simulink model "eVTOL"  (R2025b)
settings: Solver=ode45  StartTime=0.0  StopTime=7  MaxStep=1e-4  RelTol=1e-3
InitFcn:
  | load('inner_controller_design.mat')
  | load('outer_controller_design.mat')
  | load('speed_controller_design.mat')
  | load('position_controller_design.mat')
  | load('tita_controller_design.mat')
values from neighbouring files (symbols this model uses):
  b = 1e-4    (= 0.0001)    [LE_final.m]    (also in outer_controller_design.mat)
  denC = [Kc*Tcontrolador,1]    [LI_final.m]    (also in inner_controller_design.mat = [0.0127388535032 1])
  J_motor = 0.01*(0.432^2)*2    (= 0.00373248)    [LE_final.m]    (also in outer_controller_design.mat)
  J_xz = 3.25    [angular_speed_controller_design.mat]    (also in tita_controller_design.mat = 2.16666666667)
  K_pos_den = [1 2.17655923708]    [position_controller_design.mat]
  K_pos_num = [0 1.57913670417]    [position_controller_design.mat]
  Ke = 1 / Kv_rad_per_V    (= 0.0347247148564)    [LE_final.m]    (also in outer_controller_design.mat)
  KF = 0.000504745724606    [speed_controller_design.mat]
  Ki = K * z    [LE_final.m]    (also in outer_controller_design.mat = 13312.7522358)
  Kp = K    [LE_final.m]    (also in outer_controller_design.mat = 52.8005114253)
  kQ = alpha_rpm * rpm2rad^-2    (= 1.07603097028e-05)    [LE_final.m]    (also in outer_controller_design.mat)
  Kt = 1*Ke    (= 0.0347247148564)    [LE_final.m]    (also in outer_controller_design.mat)
  Ktita_den = [1 61.1449635422]    [tita_controller_design.mat]
  Ktita_num = [1557.79440274 15875.2136603]    [tita_controller_design.mat]
  Kv_den = 1    [speed_controller_design.mat]
  Kv_num = 65.3451271947    [speed_controller_design.mat]
  l = 0.3    [speed_controller_design.mat]
  l_palanca = 0.4    [tita_controller_design.mat]
  La = 0.0004    [LI_final.m]    (also in inner_controller_design.mat)
  m = 13    [speed_controller_design.mat]
  numC = [Tcontrolador,1]    [LI_final.m]    (also in inner_controller_design.mat = [0.00398089171975 1])
  Ra = 0.066    [LI_final.m]    (also in inner_controller_design.mat)
libraries: slpidlib x5, simulink_extras x4
(part 1 of 2)
settings Model: PacingRate=0.089000  Creator=Allan  LastModifiedBy=Allan

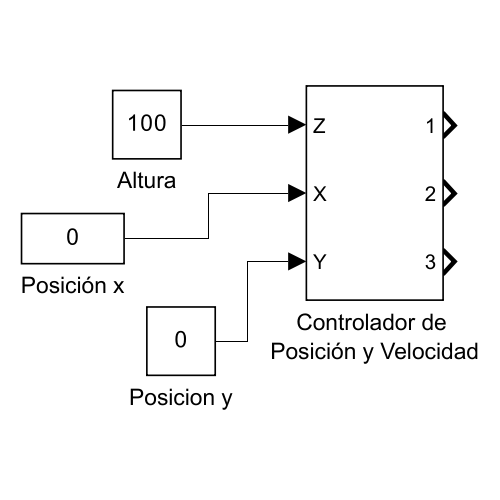
[thumbnail: Simulink's stored preview of the top-level diagram]
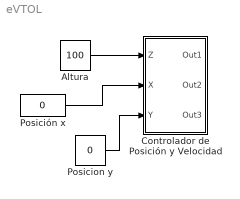
== system eVTOL ==
  Altura : Constant  Value=100
  Controlador de Posición y Velocidad : Subsystem
  Posicion y : Constant  Value=0
  Posición x : Constant  Value=0
  wires:
  Altura/1 -> Controlador de Posición y Velocidad/1(Z)
  Posición x/1 -> Controlador de Posición y Velocidad/2(X)
  Posicion y/1 -> Controlador de Posición y Velocidad/3(Y)

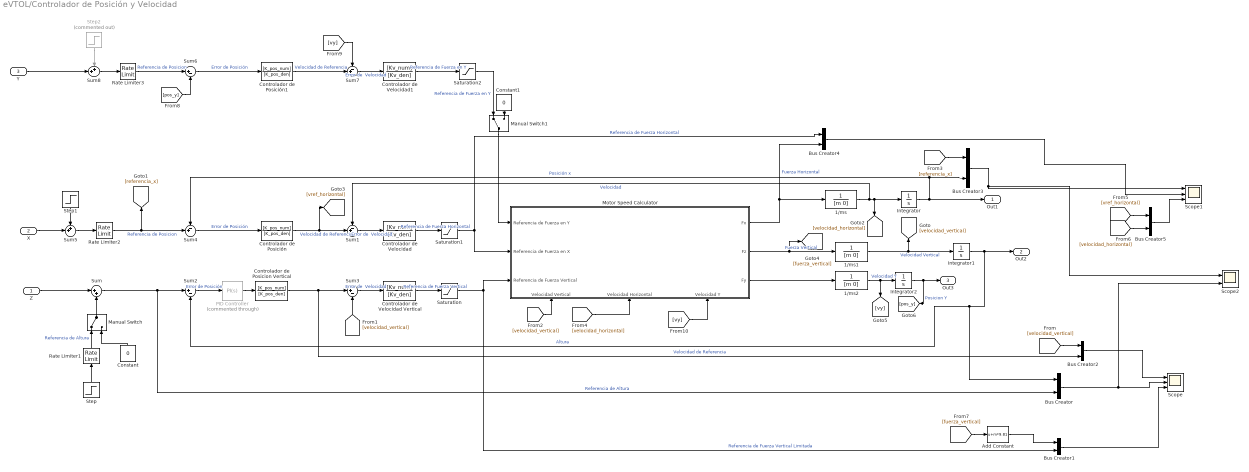
== system eVTOL/Controlador de Posición y Velocidad ==
  Z : Inport
  X : Inport  Port=2
  Y : Inport  Port=3
  1/ms : TransferFcn  Denominator=[m 0]
  1/ms1 : TransferFcn  Denominator=[m 0]
  1/ms2 : TransferFcn  Denominator=[m 0]
  Add Constant : Bias  Bias=m*9.81  SaturateOnIntegerOverflow=off
  Bus Creator{,1..5} (6 alike) : BusCreator  Inputs=2
  Constant : Constant  Value=0
  Constant1 : Constant  Value=0
  Controlador de Velocidad : TransferFcn  Numerator=[Kv_num]  Denominator=[Kv_den]
  Controlador de Velocidad1 : TransferFcn  Numerator=[Kv_num]  Denominator=[Kv_den]
  Controlador de Posicion Vertical : TransferFcn  Numerator=[K_pos_num]  Denominator=[K_pos_den]
  Controlador de Posición : TransferFcn  Numerator=[K_pos_num]  Denominator=[K_pos_den]
  Controlador de Posición1 : TransferFcn  Numerator=[K_pos_num]  Denominator=[K_pos_den]
  Controlador de Velocidad Vertical : TransferFcn  Numerator=[Kv_num]  Denominator=[Kv_den]
  Integrator : Integrator
  Integrator1 : Integrator  InitialCondition=100
  Integrator2 : Integrator
  Manual Switch : ManualSwitch
  Manual Switch1 : ManualSwitch
  Motor Speed Calculator : Subsystem
      settings: PortSchema="{\"entries\":[{\"content\":{\"sides\":[{\"content\":{\"connectorIds\":[\"In1\",\"In2\",\"In3\"]},\"type\":\"ConnectorPlacement.EquallySpacedRectSide\",\"uuid\":\"7b759047-1fb7-4341-8a14-a3cb95641d34\"},{\"content\":{\"connectorIds\":[\"Out1\",\"Out2\",\"Out3\"],\"side\":\"RIGHT\"},\"type\":\"ConnectorPlacement.EquallySpacedRectSide\",\"uuid\":\"2a3f944b-70ea-4cc6-8a8c-2d0c7e75b016\"},{\"content\":{\"side\":\"TOP\"},\"type\":\"ConnectorPlacement.EquallySpacedRectSide\",\"uuid\":\"5d8f49a3-64b1-4126-af97-ef65cef9ee4f\"},{\"content\":{\"connectorIds\":[\"In4\",\"In5\",\"In6\"],\"side\":\"BOTTOM\"},\"type\":\"ConnectorPlacement.EquallySpacedRectSide\",\"uuid\":\"3a67fbcc-1ab1-41a0-8583-aff8280d6eaa\"}]},\"type\":\"ConnectorPlacement.EquallySpacedConnector\",\"uuid\":\"910e2bb6-9332-485b-94fd-5d2df90e8b0c\"}],\"packageUris\":[\"http://schema.mathworks.com/mf0/Connector/R2020b\"],\"version\":\"1.0\"}"
  PID Controller : slpidlib/PID Controller  Commented=through  Controller=PI  Form=Parallel  TimeDomain=Continuous-time  UseExternalTs=off  SampleTime=-1  IntegratorMethod=Forward Euler  FilterMethod=Forward Euler  ControllerParametersSource=internal  P=4.353  I=6.317  UseKiTs=off  D=0  UseExternalDerivativeSource=off  N=100  UseFilter=on  TunerSelectOption=Transfer Function Based (PID Tuner App)  InitialConditionSource=internal  InitialConditionForIntegrator=0  InitialConditionForFilter=0  DifferentiatorICPrevScaledInput=0  ExternalReset=none  TrackingMode=off  Kt=1  LimitOutput=on  SatLimitsSource=internal  UpperSaturationLimit=inf  LowerSaturationLimit=-inf  LinearizeAsGain=on  AntiWindupMode=clamping  Kb=1  LimitIntegrator=off  UpperIntegratorSaturationLimit=inf  LowerIntegratorSaturationLimit=-inf  POutMin=[]  POutMax=[]  IOutMin=[]  IOutMax=[]  DOutMin=[]  DOutMax=[]  NOutMin=[]  NOutMax=[]  SumOutMin=[]  SumOutMax=[]  SaturationOutMin=[]  SaturationOutMax=[]  PParamMin=[]  PParamMax=[]  IParamMin=[]  IParamMax=[]  DParamMin=[]  DParamMax=[]  NParamMin=[]  NParamMax=[]  KbParamMin=[]  KbParamMax=[]  KtParamMin=[]  KtParamMax=[]  KbOutMin=[]  KbOutMax=[]  KtOutMin=[]  KtOutMax=[]  IntegratorOutMin=[]  IntegratorOutMax=[]  FilterOutMin=[]  FilterOutMax=[]  SumI1OutMin=[]  SumI1OutMax=[]  SumI2OutMin=[]  SumI2OutMax=[]  SumI3OutMin=[]  SumI3OutMax=[]  SumI4OutMin=[]  SumI4OutMax=[]  SumDOutMin=[]  SumDOutMax=[]  DifferentiatorOutMin=[]  DifferentiatorOutMax=[]  FilterDiffOutCoefMin=[]  FilterDiffOutCoefMax=[]  ReciprocalOutMin=[]  ReciprocalOutMax=[]  SumDenOutMin=[]  SumDenOutMax=[]  SumNumOutMin=[]  SumNumOutMax=[]  DivideOutMin=[]  DivideOutMax=[]  UdiffTsProdOutMin=[]  UdiffTsProdOutMax=[]  NTsProdOutMin=[]  NTsProdOutMax=[]  UintegralTsProdOutMin=[]  UintegralTsProdOutMax=[]  UngainTsProdOutMin=[]  UngainTsProdOutMax=[]  ClampingZeroOutDataTypeStr=Inherit: Inherit via back propagation  ClampingZeroOutMin=[]  ClampingZeroOutMax=[]  FilterDenConstantOutDataTypeStr=Inherit: Inherit via back propagation  FilterDenConstantOutMin=[]  FilterDenConstantOutMax=[]  PCopyOutDataTypeStr=Inherit: Inherit via back propagation  PCopyOutMin=[]  PCopyOutMax=[]  NCopyOutDataTypeStr=Inherit: Inherit via back propagation  NCopyOutMin=[]  NCopyOutMax=[]  IntegratorContinuousStateAttributes=''  IntegratorStateMustResolveToSignalObject=off  IntegratorRTWStateStorageClass=Auto  FilterContinuousStateAttributes=''  FilterStateMustResolveToSignalObject=off  FilterRTWStateStorageClass=Auto  ParallelPVariant=InternalParameters  IdealPVariant=Disabled  IVariant=InternalParameters  DVariant=Disabled  IntegratorVariant=Continuous  SatVariant=Enabled  AWVariant=ContClampingParallel  PCopyVariant=Disabled  TRVariant=Disabled  FdbkBlocksVariant=Forward  IdealPFdbkVariant=Disabled  SatFdbkVariant=Disabled  DerivativeFilterVariant=Disabled  NVariant=Disabled  NCopyVariant=Disabled_SignalSpec  FilterICVariant=Disabled  IntegratorICVariant=InternalICs  ExternalResetVariant=Disabled  TRSumVariant=Passthrough  SumFdbkVariant=Disabled  SumVariant=Sum_PI  TsampFilterVariant=InternalTs  TsampNgainVariant=Passthrough  TsampIntegralVariant=Disabled_SignalSpec  ExternalSaturationOutDataTypeStr=Inherit: Same as second input  DerivativeSourceVariant=Disabled  PreIntVariant=InternalPreInt
  Rate Limiter1 : RateLimiter  RisingSlewLimit=5  FallingSlewLimit=-5  SampleTimeMode=inherited  LinearizeAsGain=off
  Rate Limiter2 : RateLimiter  RisingSlewLimit=5  FallingSlewLimit=-5  SampleTimeMode=inherited  LinearizeAsGain=off
  Rate Limiter3 : RateLimiter  RisingSlewLimit=2  FallingSlewLimit=-2  SampleTimeMode=inherited  LinearizeAsGain=off
  Saturation : Saturate  UpperLimit=1.6*m*9.81  LowerLimit=0.4*m*9.81
  Saturation1 : Saturate  UpperLimit=0.2*m*9.81  LowerLimit=-0.2*m*9.81
  Saturation2 : Saturate  UpperLimit=0.5*m*9.81  LowerLimit=-0.5*m*9.81
  Scope : Scope  NumInputPorts=3
      settings: ActiveDisplayYMinimum=97.035286958696958  ActiveDisplayYMaximum=105.88496811570035  DataLoggingVariableName=ScopeData2
  Scope1 : Scope  NumInputPorts=3
      settings: ActiveDisplayYMinimum=-1.0400119613662664  ActiveDisplayYMaximum=9.3601076522964  DataLoggingVariableName=ScopeData6
  Scope2 : Scope  NumInputPorts=2
      settings: ActiveDisplayYMinimum=-0.12959032213957208  ActiveDisplayYMaximum=1.1663128992561491  DataLoggingVariableName=ScopeData7
  Step : Step  After=5  SampleTime=0
  Step1 : Step  SampleTime=0
  Step2 : Step  Commented=on  After=4  SampleTime=0
  Sum : Sum  Inputs=|++
  Sum1 : Sum  Inputs=-+|
  Sum2 : Sum  Inputs=|+-
  Sum3 : Sum  Inputs=|+-
  Sum4 : Sum  Inputs=-+|
  Sum5 : Sum  Inputs=++|
  Sum6 : Sum  Inputs=|+-
  Sum7 : Sum  Inputs=-+|
  Sum8 : Sum  Inputs=++|
  Out1 : Outport
  Out2 : Outport  Port=2
  Out3 : Outport  Port=3
  wires:
  Controlador de Posición/1 -> [vref_horizontal], Sum1/2  "Velocidad de Referencia"
  Sum4/1 -> Controlador de Posición/1  "Error de Posición"
  Sum1/1 -> Controlador de Velocidad/1  "Error de  Velocidad"
  1/ms/1 -> [velocidad_horizontal], Integrator/1, Sum1/1  "Velocidad"
  Integrator/1 -> Out1/1, Sum4/1, Bus Creator3/2  "Posición x"
  Integrator1/1 -> Sum2/2, Bus Creator/1, Out2/1  "Altura"
  Sum3/1 -> Controlador de Velocidad Vertical/1  "Error de  Velocidad"
  Sum2/1 -> PID Controller/1  "Error de Posición"
  1/ms1/1 -> [velocidad_vertical], Integrator1/1  "Velocidad Vertical"
  Controlador de Posicion Vertical/1 -> Sum3/1, Bus Creator2/2  "Velocidad de Referencia"
  Controlador de Velocidad/1 -> Saturation1/1  "Referencia de Fuerza Horizontal"
  Rate Limiter2/1 -> Sum4/2, [referencia_x]  "Referencia de Posicion"
  Sum/1 -> Bus Creator/2, Sum2/1  "Referencia de Altura"
  Motor Speed Calculator/1(Fx) -> Bus Creator4/2, 1/ms/1  "Fuerza Horizontal"
  Motor Speed Calculator/2(Fz) -> [fuerza_vertical], 1/ms1/1  "Fuerza Vertical"
  Step/1 -> Rate Limiter1/1
  Z/1 -> Sum/1
  Bus Creator/1 -> Scope2/2, Scope/2
  Bus Creator1/1 -> Scope/3
  Saturation/1 -> Motor Speed Calculator/3(Referencia de Fuerza Vertical), Bus Creator1/2  "Referencia de Fuerza Vertical Limitada"
  Saturation1/1 -> Bus Creator4/1, Motor Speed Calculator/2(Referencia de Fuerza en X)  "Referencia de Fuerza Horizontal"
  Bus Creator2/1 -> Scope/1
  Controlador de Velocidad Vertical/1 -> Saturation/1  "Referencia de Fuerza Vertical"
  [velocidad_vertical] -> Bus Creator2/1
  [velocidad_vertical] -> Sum3/2
  [velocidad_vertical] -> Motor Speed Calculator/4(Velocidad Vertical)
  Add Constant/1 -> Bus Creator1/1
  PID Controller/1 -> Controlador de Posicion Vertical/1
  Step1/1 -> Sum5/1
  X/1 -> Sum5/2
  Sum5/1 -> Rate Limiter2/1
  [referencia_x] -> Bus Creator3/1
  Bus Creator3/1 -> Scope2/1, Scope1/1
  [velocidad_horizontal] -> Motor Speed Calculator/5(Velocidad Horizontal)
  Bus Creator4/1 -> Scope1/2
  [velocidad_horizontal] -> Bus Creator5/2
  [vref_horizontal] -> Bus Creator5/1
  Bus Creator5/1 -> Scope1/3
  Sum6/1 -> Controlador de Posición1/1  "Error de Posición"
  Controlador de Velocidad1/1 -> Saturation2/1  "Referencia de Fuerza en Y"
  Controlador de Posición1/1 -> Sum7/2  "Velocidad de Referencia"
  Sum7/1 -> Controlador de Velocidad1/1  "Error de  Velocidad"
  [fuerza_vertical] -> Add Constant/1
  Motor Speed Calculator/3(Fy) -> 1/ms2/1
  1/ms2/1 -> Integrator2/1, [vy]  "Velocidad Y"
  Integrator2/1 -> [pos_y], Out3/1  "Posicion Y"
  [pos_y] -> Sum6/2
  [vy] -> Sum7/1
  Step2/1 -> Sum8/1
  Sum8/1 -> Rate Limiter3/1
  Y/1 -> Sum8/2
  Rate Limiter3/1 -> Sum6/1  "Referencia de Posicion"
  [vy] -> Motor Speed Calculator/6(Velocidad Y)
  Rate Limiter1/1 -> Manual Switch/1  "Referencia de Altura"
  Manual Switch/1 -> Sum/2
  Constant/1 -> Manual Switch/2
  Saturation2/1 -> Manual Switch1/1  "Referencia de Fuerza en Y"
  Manual Switch1/1 -> Motor Speed Calculator/1(Referencia de Fuerza en Y)
  Constant1/1 -> Manual Switch1/2

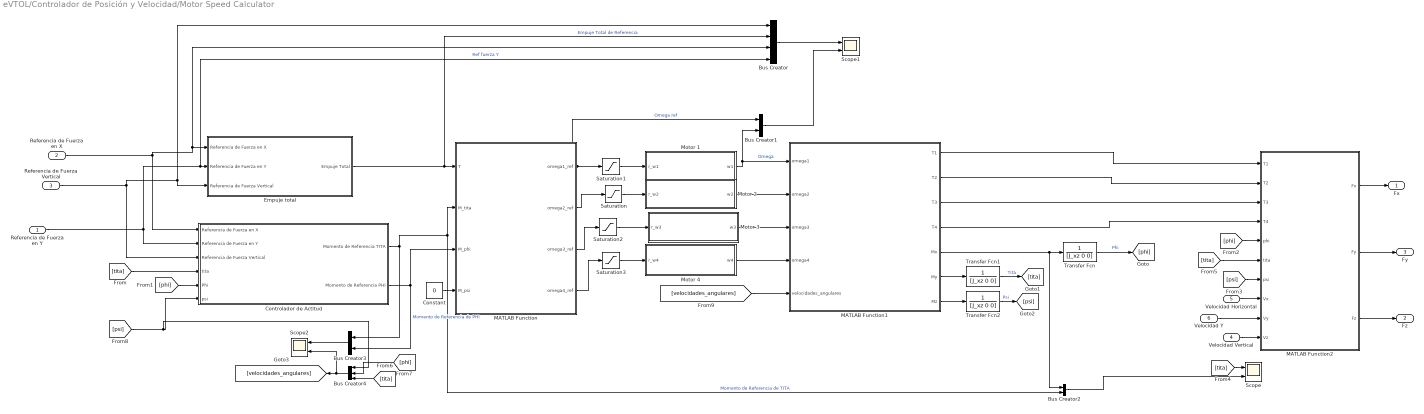
== system eVTOL/Controlador de Posición y Velocidad/Motor Speed Calculator ==
  Referencia de Fuerza en Y : Inport
  Referencia de Fuerza en X : Inport  Port=2
  Referencia de Fuerza Vertical : Inport  Port=3
  Velocidad Vertical : Inport  Port=4
  Velocidad Horizontal : Inport  Port=5
  Velocidad Y : Inport  Port=6
  Bus Creator : BusCreator  Inputs=4
  Bus Creator1 : BusCreator  Inputs=2
  Bus Creator2 : BusCreator  Inputs=2
  Bus Creator3 : BusCreator  Inputs=2
  Bus Creator4 : BusCreator  Inputs=3
  Constant : Constant  Value=0
  Controlador de Actitud : Subsystem
  Empuje total : Subsystem
  MATLAB Function : MATLAB Function  TreatAsAtomicUnit=on
  MATLAB Function1 : MATLAB Function  TreatAsAtomicUnit=on
  MATLAB Function2 : MATLAB Function  TreatAsAtomicUnit=on
  Motor 1 : Subsystem
  Motor 2 : Subsystem
  Motor 3 : Subsystem
  Motor 4 : Subsystem
  Saturation{,1..3} (4 alike) : Saturate  UpperLimit=350  LowerLimit=0
  Scope : Scope  NumInputPorts=2
      settings: ActiveDisplayYMinimum=-22.318577397264981  ActiveDisplayYMaximum=3.461658790222101  DataLoggingVariableName=ScopeData3
  Scope1 : Scope  NumInputPorts=2
      settings: ActiveDisplayYMinimum=-65.605934542157769  ActiveDisplayYMaximum=245.78377582447797  DataLoggingVariableName=ScopeData4
  Scope2 : Scope  NumInputPorts=2
      settings: ActiveDisplayYMinimum=-3.75  ActiveDisplayYMaximum=3.75  DataLoggingVariableName=ScopeData9
  Transfer Fcn : TransferFcn  Denominator=[J_xz 0 0]
  Transfer Fcn1 : TransferFcn  Denominator=[J_xz 0 0]
  Transfer Fcn2 : TransferFcn  Denominator=[J_xz 0 0]
  Fx : Outport  VectorParamsAs1DForOutWhenUnconnected=off
  Fz : Outport  Port=2  VectorParamsAs1DForOutWhenUnconnected=off
  Fy : Outport  Port=3  VectorParamsAs1DForOutWhenUnconnected=off
  wires:
  Referencia de Fuerza en X/1 -> Bus Creator/3, Empuje total/1(Referencia de Fuerza en X), Controlador de Actitud/1(Referencia de Fuerza en X)
  Referencia de Fuerza Vertical/1 -> Bus Creator/1, Empuje total/3(Referencia de Fuerza Vertical), Controlador de Actitud/3(Referencia de Fuerza Vertical)
  Empuje total/1(Empuje Total) -> Bus Creator/2, MATLAB Function/1(T)  "Empuje Total de Referencia"
  MATLAB Function/1(omega1_ref) -> Saturation1/1, Bus Creator1/1  "Omega ref"
  Motor 1/1(w1) -> Bus Creator1/2, MATLAB Function1/1(omega1)  "Omega"
  Motor 2/1(w2) -> MATLAB Function1/2(omega2)
  MATLAB Function1/1(T1) -> MATLAB Function2/1(T1)
  Transfer Fcn/1 -> [phi]  "Phi"
  MATLAB Function2/3(Fz) -> Fz/1
  MATLAB Function2/1(Fx) -> Fx/1
  Bus Creator/1 -> Scope1/1
  Bus Creator1/1 -> Scope1/2
  MATLAB Function/2(omega2_ref) -> Saturation/1
  [tita] -> Controlador de Actitud/4(tita)
  Saturation/1 -> Motor 2/1(r_w2)
  Saturation1/1 -> Motor 1/1(r_w1)
  Controlador de Actitud/1(Momento de Referencia TITA) -> Bus Creator2/2, MATLAB Function/2(M_tita), Bus Creator3/1  "Momento de Referencia de TITA"
  Bus Creator2/1 -> Scope/2
  Referencia de Fuerza en Y/1 -> Controlador de Actitud/2(Referencia de Fuerza en Y), Bus Creator/4, Empuje total/2(Referencia de Fuerza en Y)  "Ref fuerza Y"
  Controlador de Actitud/2(Momento de Referencia PHI) -> MATLAB Function/3(M_phi), Bus Creator3/2  "Momento de Referencia de PHI"
  Saturation2/1 -> Motor 3/1(r_w3)
  Saturation3/1 -> Motor 4/1(r_w4)
  MATLAB Function/3(omega3_ref) -> Saturation2/1
  MATLAB Function/4(omega4_ref) -> Saturation3/1
  Motor 3/1(w3) -> MATLAB Function1/3(omega3)
  Motor 4/1(w4) -> MATLAB Function1/4(omega4)
  Constant/1 -> MATLAB Function/4(M_psi)
  MATLAB Function1/5(Mx) -> Bus Creator2/1, Transfer Fcn/1
  MATLAB Function1/6(My) -> Transfer Fcn1/1
  Transfer Fcn1/1 -> [tita]  "Tita"
  MATLAB Function1/7(Mz) -> Transfer Fcn2/1
  [phi] -> Controlador de Actitud/5(Phi)
  MATLAB Function2/2(Fy) -> Fy/1
  Velocidad Vertical/1 -> MATLAB Function2/10(Vz)
  Velocidad Horizontal/1 -> MATLAB Function2/8(Vx)
  Velocidad Y/1 -> MATLAB Function2/9(Vy)
  [phi] -> MATLAB Function2/5(phi)
  Transfer Fcn2/1 -> [psi]  "Psi"
  [psi] -> MATLAB Function2/7(psi)
  [tita] -> Scope/1
  [tita] -> MATLAB Function2/6(tita)
  [phi] -> Bus Creator4/2
  [tita] -> Bus Creator4/3
  Bus Creator3/1 -> Scope2/1
  Bus Creator4/1 -> Scope2/2, [velocidades_angulares]
  MATLAB Function1/2(T2) -> MATLAB Function2/2(T2)
  MATLAB Function1/3(T3) -> MATLAB Function2/3(T3)
  MATLAB Function1/4(T4) -> MATLAB Function2/4(T4)
  [psi] -> Bus Creator4/1, Controlador de Actitud/6(psi)
  [velocidades_angulares] -> MATLAB Function1/5(velocidades_angulares)

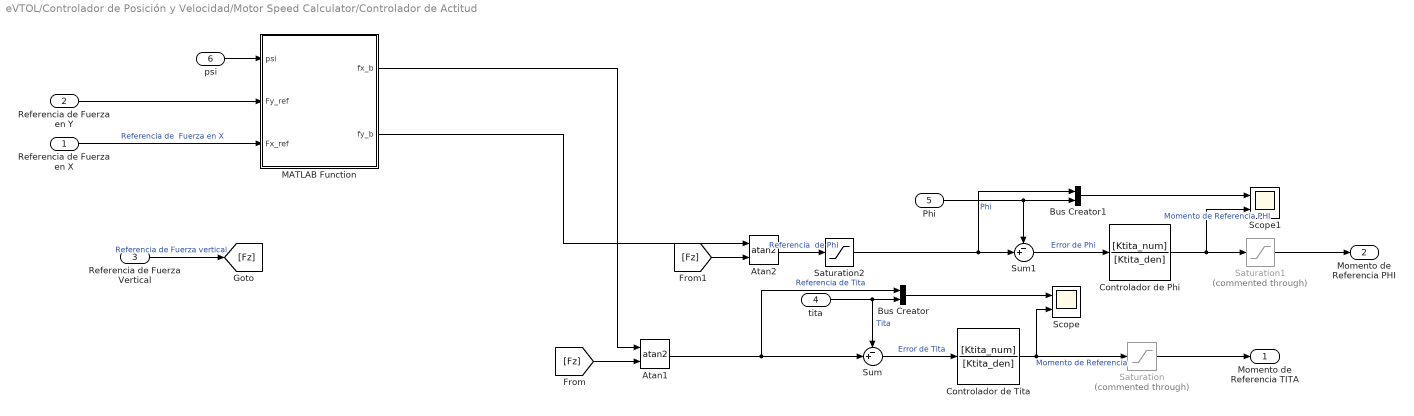
== system eVTOL/Controlador de Posición y Velocidad/Motor Speed Calculator/Controlador de Actitud ==
  Referencia de Fuerza en X : Inport
  Referencia de Fuerza en Y : Inport  Port=2
  Referencia de Fuerza Vertical : Inport  Port=3
  tita : Inport  Port=4
  Phi : Inport  Port=5
  psi : Inport  Port=6
  Atan1 : Trigonometry  Operator=atan2
  Atan2 : Trigonometry  Operator=atan2
  Bus Creator : BusCreator  Inputs=2
  Bus Creator1 : BusCreator  Inputs=2
  Controlador de Phi : TransferFcn  Numerator=[Ktita_num]  Denominator=[Ktita_den]
  Controlador de Tita : TransferFcn  Numerator=[Ktita_num]  Denominator=[Ktita_den]
  MATLAB Function : MATLAB Function  TreatAsAtomicUnit=on
  Saturation : Saturate  Commented=through  UpperLimit=3  LowerLimit=-3
  Saturation1 : Saturate  Commented=through  UpperLimit=3  LowerLimit=-3
  Saturation2 : Saturate  UpperLimit=30*pi/180  LowerLimit=-30*pi/180
  Scope : Scope  NumInputPorts=2
      settings: ActiveDisplayYMinimum=-0.99160938377445429  ActiveDisplayYMaximum=0.84856838437054594  DataLoggingVariableName=ScopeData5
  Scope1 : Scope  NumInputPorts=2
      settings: ActiveDisplayYMinimum=3.1274545211722726  ActiveDisplayYMaximum=3.153212088221645  DataLoggingVariableName=ScopeData8
  Sum : Sum  Inputs=-+|
  Sum1 : Sum  Inputs=-+|
  Momento de Referencia TITA : Outport
  Momento de Referencia PHI : Outport  Port=2
  wires:
  tita/1 -> Sum/1, Bus Creator/2  "Tita"
  Controlador de Tita/1 -> Saturation/1, Scope/2  "Momento de Referencia"
  Sum/1 -> Controlador de Tita/1  "Error de Tita"
  Bus Creator/1 -> Scope/1
  Atan1/1 -> Sum/2, Bus Creator/1  "Referencia de Tita"
  Sum1/1 -> Controlador de Phi/1  "Error de Phi"
  Controlador de Phi/1 -> Saturation1/1, Scope1/2  "Momento de Referencia PHI"
  Atan2/1 -> Saturation2/1  "Referencia  de Phi"
  Phi/1 -> Sum1/1, Bus Creator1/2  "Phi"
  Bus Creator1/1 -> Scope1/1
  Referencia de Fuerza Vertical/1 -> [Fz]  "Referencia de Fuerza vertical"
  MATLAB Function/1(fx_b) -> Atan1/1
  [Fz] -> Atan1/2
  Saturation/1 -> Momento de Referencia TITA/1
  Saturation1/1 -> Momento de Referencia PHI/1
  Referencia de Fuerza en Y/1 -> MATLAB Function/2(Fy_ref)
  Referencia de Fuerza en X/1 -> MATLAB Function/3(Fx_ref)  "Referencia de  Fuerza en X"
  psi/1 -> MATLAB Function/1(psi)
  Saturation2/1 -> Sum1/2, Bus Creator1/1
  MATLAB Function/2(fy_b) -> Atan2/1
  [Fz] -> Atan2/2

== system eVTOL/Controlador de Posición y Velocidad/Motor Speed Calculator/Empuje total ==
  Referencia de Fuerza en X : Inport
  Referencia de Fuerza en Y : Inport  Port=2
  Referencia de Fuerza Vertical : Inport  Port=3
  Dot Product : DotProduct  OutDataTypeStr=Inherit: Inherit via internal rule
  Dot Product1 : DotProduct  OutDataTypeStr=Inherit: Inherit via internal rule
  Dot Product2 : DotProduct  OutDataTypeStr=Inherit: Inherit via internal rule
  Sqrt : Sqrt
  Sum : Sum  Inputs=|+++
  Empuje Total : Outport
  wires:
  Dot Product/1 -> Sum/2
  Referencia de Fuerza Vertical/1 -> Dot Product/2, Dot Product/1
  Referencia de Fuerza en X/1 -> Dot Product1/2, Dot Product1/1
  Sum/1 -> Sqrt/1
  Sqrt/1 -> Empuje Total/1  "Empuje  Total"
  Dot Product1/1 -> Sum/1
  Referencia de Fuerza en Y/1 -> Dot Product2/2, Dot Product2/1
  Dot Product2/1 -> Sum/3

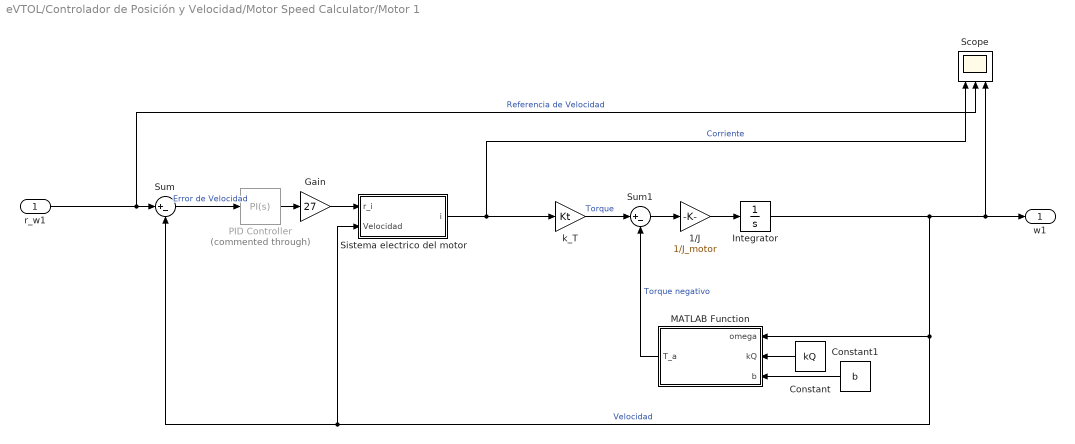
== system eVTOL/Controlador de Posición y Velocidad/Motor Speed Calculator/Motor 1 ==
  r_w1 : Inport
  1/J : Gain  Gain=1/J_motor
  Constant : Constant  Value=kQ
  Constant1 : Constant  Value=b
  Gain : Gain  Gain=27
  Integrator : Integrator  InitialCondition=181
  MATLAB Function : MATLAB Function  TreatAsAtomicUnit=on
  PID Controller : slpidlib/PID Controller  Commented=through  Controller=PI  Form=Parallel  TimeDomain=Continuous-time  UseExternalTs=off  SampleTime=-1  IntegratorMethod=Forward Euler  FilterMethod=Forward Euler  ControllerParametersSource=internal  P=Kp  I=Ki  UseKiTs=off  D=0  UseExternalDerivativeSource=off  N=0  UseFilter=on  TunerSelectOption=Transfer Function Based (PID Tuner App)  InitialConditionSource=internal  InitialConditionForIntegrator=0  InitialConditionForFilter=0  DifferentiatorICPrevScaledInput=0  ExternalReset=none  TrackingMode=off  Kt=1  LimitOutput=off  SatLimitsSource=internal  UpperSaturationLimit=150  LowerSaturationLimit=0  LinearizeAsGain=on  AntiWindupMode=none  Kb=0.2  LimitIntegrator=off  UpperIntegratorSaturationLimit=inf  LowerIntegratorSaturationLimit=-inf  POutMin=[]  POutMax=[]  IOutMin=[]  IOutMax=[]  DOutMin=[]  DOutMax=[]  NOutMin=[]  NOutMax=[]  SumOutMin=[]  SumOutMax=[]  SaturationOutMin=[]  SaturationOutMax=[]  PParamMin=[]  PParamMax=[]  IParamMin=[]  IParamMax=[]  DParamMin=[]  DParamMax=[]  NParamMin=[]  NParamMax=[]  KbParamMin=[]  KbParamMax=[]  KtParamMin=[]  KtParamMax=[]  KbOutMin=[]  KbOutMax=[]  KtOutMin=[]  KtOutMax=[]  IntegratorOutMin=[]  IntegratorOutMax=[]  FilterOutMin=[]  FilterOutMax=[]  SumI1OutMin=[]  SumI1OutMax=[]  SumI2OutMin=[]  SumI2OutMax=[]  SumI3OutMin=[]  SumI3OutMax=[]  SumI4OutMin=[]  SumI4OutMax=[]  SumDOutMin=[]  SumDOutMax=[]  DifferentiatorOutMin=[]  DifferentiatorOutMax=[]  FilterDiffOutCoefMin=[]  FilterDiffOutCoefMax=[]  ReciprocalOutMin=[]  ReciprocalOutMax=[]  SumDenOutMin=[]  SumDenOutMax=[]  SumNumOutMin=[]  SumNumOutMax=[]  DivideOutMin=[]  DivideOutMax=[]  UdiffTsProdOutMin=[]  UdiffTsProdOutMax=[]  NTsProdOutMin=[]  NTsProdOutMax=[]  UintegralTsProdOutMin=[]  UintegralTsProdOutMax=[]  UngainTsProdOutMin=[]  UngainTsProdOutMax=[]  ClampingZeroOutDataTypeStr=Inherit: Inherit via back propagation  ClampingZeroOutMin=[]  ClampingZeroOutMax=[]  FilterDenConstantOutDataTypeStr=Inherit: Inherit via back propagation  FilterDenConstantOutMin=[]  FilterDenConstantOutMax=[]  PCopyOutDataTypeStr=Inherit: Inherit via back propagation  PCopyOutMin=[]  PCopyOutMax=[]  NCopyOutDataTypeStr=Inherit: Inherit via back propagation  NCopyOutMin=[]  NCopyOutMax=[]  IntegratorContinuousStateAttributes=''  IntegratorStateMustResolveToSignalObject=off  IntegratorRTWStateStorageClass=Auto  FilterContinuousStateAttributes=''  FilterStateMustResolveToSignalObject=off  FilterRTWStateStorageClass=Auto  ParallelPVariant=InternalParameters  IdealPVariant=Disabled  IVariant=InternalParameters  DVariant=Disabled  IntegratorVariant=Continuous  SatVariant=Disabled  AWVariant=Passthrough  PCopyVariant=Disabled  TRVariant=Disabled  FdbkBlocksVariant=Forward  IdealPFdbkVariant=Disabled  SatFdbkVariant=Disabled  DerivativeFilterVariant=Disabled  NVariant=Disabled  NCopyVariant=Disabled_SignalSpec  FilterICVariant=Disabled  IntegratorICVariant=InternalICs  ExternalResetVariant=Disabled  TRSumVariant=Passthrough  SumFdbkVariant=Disabled  SumVariant=Sum_PI  TsampFilterVariant=InternalTs  TsampNgainVariant=Passthrough  TsampIntegralVariant=Disabled_SignalSpec  ExternalSaturationOutDataTypeStr=Inherit: Same as second input  DerivativeSourceVariant=Disabled  PreIntVariant=InternalPreInt
  Scope : Scope  NumInputPorts=3
      settings: ActiveDisplayYMinimum=-43.749999999999993  ActiveDisplayYMaximum=393.75
  Sistema electrico del motor : Subsystem
  Sum : Sum  Inputs=|+-
  Sum1 : Sum  Inputs=|+-
  k_T : Gain  Gain=Kt
  w1 : Outport
  wires:
  k_T/1 -> Sum1/1  "Torque"
  Sum/1 -> PID Controller/1  "Error de Velocidad"
  MATLAB Function/1(T_a) -> Sum1/2  "Torque negativo"
  1/J/1 -> Integrator/1
  Constant/1 -> MATLAB Function/2(kQ)
  Sum1/1 -> 1/J/1
  Integrator/1 -> w1/1, Scope/3, MATLAB Function/1(omega), Sum/2, Sistema electrico del motor/2(Velocidad)  "Velocidad"
  Constant1/1 -> MATLAB Function/3(b)
  r_w1/1 -> Scope/2, Sum/1  "Referencia de Velocidad"
  Sistema electrico del motor/1(i) -> k_T/1, Scope/1  "Corriente"
  PID Controller/1 -> Gain/1
  Gain/1 -> Sistema electrico del motor/1(r_i)

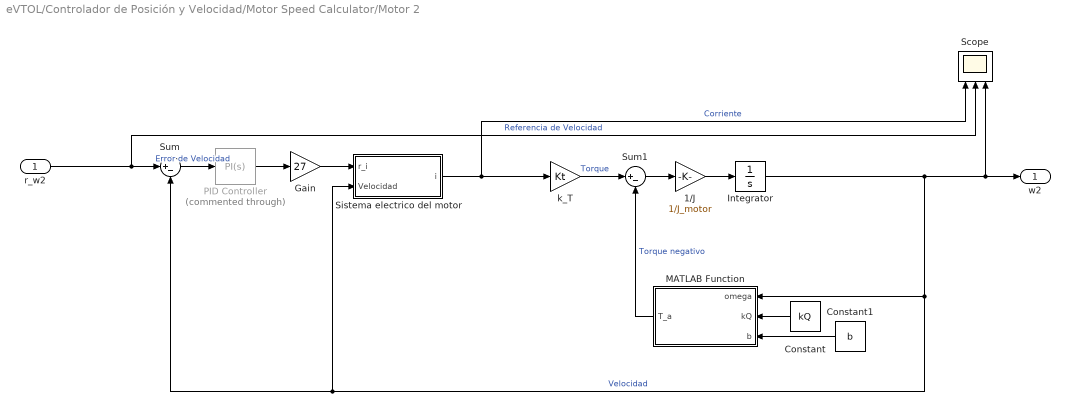
== system eVTOL/Controlador de Posición y Velocidad/Motor Speed Calculator/Motor 2 ==
  r_w2 : Inport
  1/J : Gain  Gain=1/J_motor
  Constant : Constant  Value=kQ
  Constant1 : Constant  Value=b
  Gain : Gain  Gain=27
  Integrator : Integrator  InitialCondition=181
  MATLAB Function : MATLAB Function  TreatAsAtomicUnit=on
  PID Controller : slpidlib/PID Controller  Commented=through  Controller=PI  Form=Parallel  TimeDomain=Continuous-time  UseExternalTs=off  SampleTime=-1  IntegratorMethod=Forward Euler  FilterMethod=Forward Euler  ControllerParametersSource=internal  P=Kp  I=Ki  UseKiTs=off  D=0  UseExternalDerivativeSource=off  N=0  UseFilter=on  TunerSelectOption=Transfer Function Based (PID Tuner App)  InitialConditionSource=internal  InitialConditionForIntegrator=0  InitialConditionForFilter=0  DifferentiatorICPrevScaledInput=0  ExternalReset=none  TrackingMode=off  Kt=1  LimitOutput=off  SatLimitsSource=internal  UpperSaturationLimit=150  LowerSaturationLimit=0  LinearizeAsGain=on  AntiWindupMode=none  Kb=0.2  LimitIntegrator=off  UpperIntegratorSaturationLimit=inf  LowerIntegratorSaturationLimit=-inf  POutMin=[]  POutMax=[]  IOutMin=[]  IOutMax=[]  DOutMin=[]  DOutMax=[]  NOutMin=[]  NOutMax=[]  SumOutMin=[]  SumOutMax=[]  SaturationOutMin=[]  SaturationOutMax=[]  PParamMin=[]  PParamMax=[]  IParamMin=[]  IParamMax=[]  DParamMin=[]  DParamMax=[]  NParamMin=[]  NParamMax=[]  KbParamMin=[]  KbParamMax=[]  KtParamMin=[]  KtParamMax=[]  KbOutMin=[]  KbOutMax=[]  KtOutMin=[]  KtOutMax=[]  IntegratorOutMin=[]  IntegratorOutMax=[]  FilterOutMin=[]  FilterOutMax=[]  SumI1OutMin=[]  SumI1OutMax=[]  SumI2OutMin=[]  SumI2OutMax=[]  SumI3OutMin=[]  SumI3OutMax=[]  SumI4OutMin=[]  SumI4OutMax=[]  SumDOutMin=[]  SumDOutMax=[]  DifferentiatorOutMin=[]  DifferentiatorOutMax=[]  FilterDiffOutCoefMin=[]  FilterDiffOutCoefMax=[]  ReciprocalOutMin=[]  ReciprocalOutMax=[]  SumDenOutMin=[]  SumDenOutMax=[]  SumNumOutMin=[]  SumNumOutMax=[]  DivideOutMin=[]  DivideOutMax=[]  UdiffTsProdOutMin=[]  UdiffTsProdOutMax=[]  NTsProdOutMin=[]  NTsProdOutMax=[]  UintegralTsProdOutMin=[]  UintegralTsProdOutMax=[]  UngainTsProdOutMin=[]  UngainTsProdOutMax=[]  ClampingZeroOutDataTypeStr=Inherit: Inherit via back propagation  ClampingZeroOutMin=[]  ClampingZeroOutMax=[]  FilterDenConstantOutDataTypeStr=Inherit: Inherit via back propagation  FilterDenConstantOutMin=[]  FilterDenConstantOutMax=[]  PCopyOutDataTypeStr=Inherit: Inherit via back propagation  PCopyOutMin=[]  PCopyOutMax=[]  NCopyOutDataTypeStr=Inherit: Inherit via back propagation  NCopyOutMin=[]  NCopyOutMax=[]  IntegratorContinuousStateAttributes=''  IntegratorStateMustResolveToSignalObject=off  IntegratorRTWStateStorageClass=Auto  FilterContinuousStateAttributes=''  FilterStateMustResolveToSignalObject=off  FilterRTWStateStorageClass=Auto  ParallelPVariant=InternalParameters  IdealPVariant=Disabled  IVariant=InternalParameters  DVariant=Disabled  IntegratorVariant=Continuous  SatVariant=Disabled  AWVariant=Passthrough  PCopyVariant=Disabled  TRVariant=Disabled  FdbkBlocksVariant=Forward  IdealPFdbkVariant=Disabled  SatFdbkVariant=Disabled  DerivativeFilterVariant=Disabled  NVariant=Disabled  NCopyVariant=Disabled_SignalSpec  FilterICVariant=Disabled  IntegratorICVariant=InternalICs  ExternalResetVariant=Disabled  TRSumVariant=Passthrough  SumFdbkVariant=Disabled  SumVariant=Sum_PI  TsampFilterVariant=InternalTs  TsampNgainVariant=Passthrough  TsampIntegralVariant=Disabled_SignalSpec  ExternalSaturationOutDataTypeStr=Inherit: Same as second input  DerivativeSourceVariant=Disabled  PreIntVariant=InternalPreInt
  Scope : Scope  NumInputPorts=3
      settings: ActiveDisplayYMinimum=237.40854742566631  ActiveDisplayYMaximum=324.6469636585125
  Sistema electrico del motor : Subsystem
  Sum : Sum  Inputs=|+-
  Sum1 : Sum  Inputs=|+-
  k_T : Gain  Gain=Kt
  w2 : Outport
  wires:
  k_T/1 -> Sum1/1  "Torque"
  Sum/1 -> PID Controller/1  "Error de Velocidad"
  MATLAB Function/1(T_a) -> Sum1/2  "Torque negativo"
  1/J/1 -> Integrator/1
  Constant/1 -> MATLAB Function/2(kQ)
  Sum1/1 -> 1/J/1
  Integrator/1 -> w2/1, Scope/3, MATLAB Function/1(omega), Sistema electrico del motor/2(Velocidad), Sum/2  "Velocidad"
  Constant1/1 -> MATLAB Function/3(b)
  r_w2/1 -> Scope/2, Sum/1  "Referencia de Velocidad"
  Sistema electrico del motor/1(i) -> k_T/1, Scope/1  "Corriente"
  PID Controller/1 -> Gain/1
  Gain/1 -> Sistema electrico del motor/1(r_i)

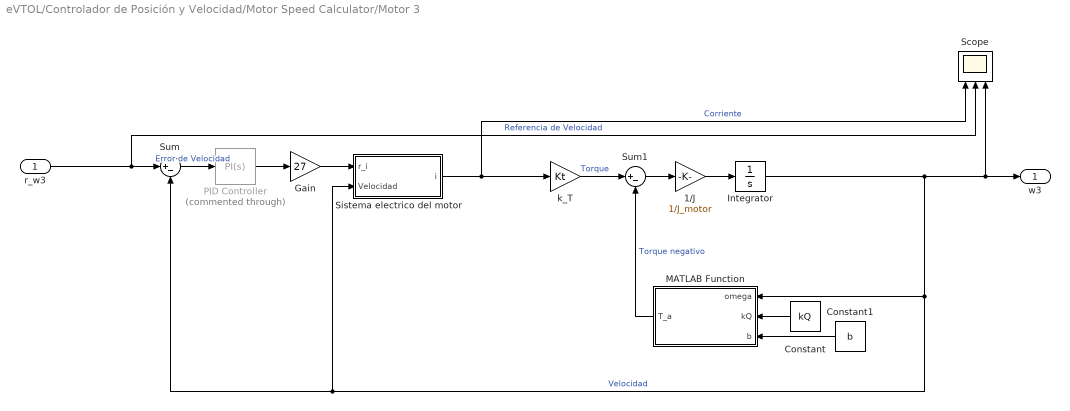
== system eVTOL/Controlador de Posición y Velocidad/Motor Speed Calculator/Motor 3 ==
  r_w3 : Inport
  1/J : Gain  Gain=1/J_motor
  Constant : Constant  Value=kQ
  Constant1 : Constant  Value=b
  Gain : Gain  Gain=27
  Integrator : Integrator  InitialCondition=181
  MATLAB Function : MATLAB Function  TreatAsAtomicUnit=on
  PID Controller : slpidlib/PID Controller  Commented=through  Controller=PI  Form=Parallel  TimeDomain=Continuous-time  UseExternalTs=off  SampleTime=-1  IntegratorMethod=Forward Euler  FilterMethod=Forward Euler  ControllerParametersSource=internal  P=Kp  I=Ki  UseKiTs=off  D=0  UseExternalDerivativeSource=off  N=0  UseFilter=on  TunerSelectOption=Transfer Function Based (PID Tuner App)  InitialConditionSource=internal  InitialConditionForIntegrator=0  InitialConditionForFilter=0  DifferentiatorICPrevScaledInput=0  ExternalReset=none  TrackingMode=off  Kt=1  LimitOutput=off  SatLimitsSource=internal  UpperSaturationLimit=150  LowerSaturationLimit=0  LinearizeAsGain=on  AntiWindupMode=none  Kb=0.2  LimitIntegrator=off  UpperIntegratorSaturationLimit=inf  LowerIntegratorSaturationLimit=-inf  POutMin=[]  POutMax=[]  IOutMin=[]  IOutMax=[]  DOutMin=[]  DOutMax=[]  NOutMin=[]  NOutMax=[]  SumOutMin=[]  SumOutMax=[]  SaturationOutMin=[]  SaturationOutMax=[]  PParamMin=[]  PParamMax=[]  IParamMin=[]  IParamMax=[]  DParamMin=[]  DParamMax=[]  NParamMin=[]  NParamMax=[]  KbParamMin=[]  KbParamMax=[]  KtParamMin=[]  KtParamMax=[]  KbOutMin=[]  KbOutMax=[]  KtOutMin=[]  KtOutMax=[]  IntegratorOutMin=[]  IntegratorOutMax=[]  FilterOutMin=[]  FilterOutMax=[]  SumI1OutMin=[]  SumI1OutMax=[]  SumI2OutMin=[]  SumI2OutMax=[]  SumI3OutMin=[]  SumI3OutMax=[]  SumI4OutMin=[]  SumI4OutMax=[]  SumDOutMin=[]  SumDOutMax=[]  DifferentiatorOutMin=[]  DifferentiatorOutMax=[]  FilterDiffOutCoefMin=[]  FilterDiffOutCoefMax=[]  ReciprocalOutMin=[]  ReciprocalOutMax=[]  SumDenOutMin=[]  SumDenOutMax=[]  SumNumOutMin=[]  SumNumOutMax=[]  DivideOutMin=[]  DivideOutMax=[]  UdiffTsProdOutMin=[]  UdiffTsProdOutMax=[]  NTsProdOutMin=[]  NTsProdOutMax=[]  UintegralTsProdOutMin=[]  UintegralTsProdOutMax=[]  UngainTsProdOutMin=[]  UngainTsProdOutMax=[]  ClampingZeroOutDataTypeStr=Inherit: Inherit via back propagation  ClampingZeroOutMin=[]  ClampingZeroOutMax=[]  FilterDenConstantOutDataTypeStr=Inherit: Inherit via back propagation  FilterDenConstantOutMin=[]  FilterDenConstantOutMax=[]  PCopyOutDataTypeStr=Inherit: Inherit via back propagation  PCopyOutMin=[]  PCopyOutMax=[]  NCopyOutDataTypeStr=Inherit: Inherit via back propagation  NCopyOutMin=[]  NCopyOutMax=[]  IntegratorContinuousStateAttributes=''  IntegratorStateMustResolveToSignalObject=off  IntegratorRTWStateStorageClass=Auto  FilterContinuousStateAttributes=''  FilterStateMustResolveToSignalObject=off  FilterRTWStateStorageClass=Auto  ParallelPVariant=InternalParameters  IdealPVariant=Disabled  IVariant=InternalParameters  DVariant=Disabled  IntegratorVariant=Continuous  SatVariant=Disabled  AWVariant=Passthrough  PCopyVariant=Disabled  TRVariant=Disabled  FdbkBlocksVariant=Forward  IdealPFdbkVariant=Disabled  SatFdbkVariant=Disabled  DerivativeFilterVariant=Disabled  NVariant=Disabled  NCopyVariant=Disabled_SignalSpec  FilterICVariant=Disabled  IntegratorICVariant=InternalICs  ExternalResetVariant=Disabled  TRSumVariant=Passthrough  SumFdbkVariant=Disabled  SumVariant=Sum_PI  TsampFilterVariant=InternalTs  TsampNgainVariant=Passthrough  TsampIntegralVariant=Disabled_SignalSpec  ExternalSaturationOutDataTypeStr=Inherit: Same as second input  DerivativeSourceVariant=Disabled  PreIntVariant=InternalPreInt
  Scope : Scope  NumInputPorts=3
      settings: ActiveDisplayYMinimum=237.40854742566631  ActiveDisplayYMaximum=324.6469636585125
  Sistema electrico del motor : Subsystem
  Sum : Sum  Inputs=|+-
  Sum1 : Sum  Inputs=|+-
  k_T : Gain  Gain=Kt
  w3 : Outport
  wires:
  k_T/1 -> Sum1/1  "Torque"
  Sum/1 -> PID Controller/1  "Error de Velocidad"
  MATLAB Function/1(T_a) -> Sum1/2  "Torque negativo"
  1/J/1 -> Integrator/1
  Constant/1 -> MATLAB Function/2(kQ)
  Sum1/1 -> 1/J/1
  Integrator/1 -> w3/1, Scope/3, MATLAB Function/1(omega), Sistema electrico del motor/2(Velocidad), Sum/2  "Velocidad"
  Constant1/1 -> MATLAB Function/3(b)
  r_w3/1 -> Scope/2, Sum/1  "Referencia de Velocidad"
  Sistema electrico del motor/1(i) -> k_T/1, Scope/1  "Corriente"
  PID Controller/1 -> Gain/1
  Gain/1 -> Sistema electrico del motor/1(r_i)

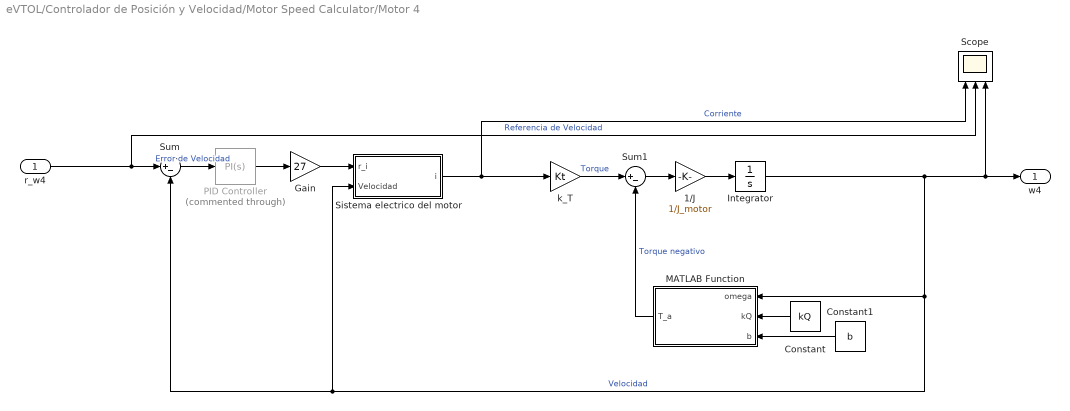
== system eVTOL/Controlador de Posición y Velocidad/Motor Speed Calculator/Motor 4 ==
  r_w4 : Inport
  1/J : Gain  Gain=1/J_motor
  Constant : Constant  Value=kQ
  Constant1 : Constant  Value=b
  Gain : Gain  Gain=27
  Integrator : Integrator  InitialCondition=181
  MATLAB Function : MATLAB Function  TreatAsAtomicUnit=on
  PID Controller : slpidlib/PID Controller  Commented=through  Controller=PI  Form=Parallel  TimeDomain=Continuous-time  UseExternalTs=off  SampleTime=-1  IntegratorMethod=Forward Euler  FilterMethod=Forward Euler  ControllerParametersSource=internal  P=Kp  I=Ki  UseKiTs=off  D=0  UseExternalDerivativeSource=off  N=0  UseFilter=on  TunerSelectOption=Transfer Function Based (PID Tuner App)  InitialConditionSource=internal  InitialConditionForIntegrator=0  InitialConditionForFilter=0  DifferentiatorICPrevScaledInput=0  ExternalReset=none  TrackingMode=off  Kt=1  LimitOutput=off  SatLimitsSource=internal  UpperSaturationLimit=150  LowerSaturationLimit=0  LinearizeAsGain=on  AntiWindupMode=none  Kb=0.2  LimitIntegrator=off  UpperIntegratorSaturationLimit=inf  LowerIntegratorSaturationLimit=-inf  POutMin=[]  POutMax=[]  IOutMin=[]  IOutMax=[]  DOutMin=[]  DOutMax=[]  NOutMin=[]  NOutMax=[]  SumOutMin=[]  SumOutMax=[]  SaturationOutMin=[]  SaturationOutMax=[]  PParamMin=[]  PParamMax=[]  IParamMin=[]  IParamMax=[]  DParamMin=[]  DParamMax=[]  NParamMin=[]  NParamMax=[]  KbParamMin=[]  KbParamMax=[]  KtParamMin=[]  KtParamMax=[]  KbOutMin=[]  KbOutMax=[]  KtOutMin=[]  KtOutMax=[]  IntegratorOutMin=[]  IntegratorOutMax=[]  FilterOutMin=[]  FilterOutMax=[]  SumI1OutMin=[]  SumI1OutMax=[]  SumI2OutMin=[]  SumI2OutMax=[]  SumI3OutMin=[]  SumI3OutMax=[]  SumI4OutMin=[]  SumI4OutMax=[]  SumDOutMin=[]  SumDOutMax=[]  DifferentiatorOutMin=[]  DifferentiatorOutMax=[]  FilterDiffOutCoefMin=[]  FilterDiffOutCoefMax=[]  ReciprocalOutMin=[]  ReciprocalOutMax=[]  SumDenOutMin=[]  SumDenOutMax=[]  SumNumOutMin=[]  SumNumOutMax=[]  DivideOutMin=[]  DivideOutMax=[]  UdiffTsProdOutMin=[]  UdiffTsProdOutMax=[]  NTsProdOutMin=[]  NTsProdOutMax=[]  UintegralTsProdOutMin=[]  UintegralTsProdOutMax=[]  UngainTsProdOutMin=[]  UngainTsProdOutMax=[]  ClampingZeroOutDataTypeStr=Inherit: Inherit via back propagation  ClampingZeroOutMin=[]  ClampingZeroOutMax=[]  FilterDenConstantOutDataTypeStr=Inherit: Inherit via back propagation  FilterDenConstantOutMin=[]  FilterDenConstantOutMax=[]  PCopyOutDataTypeStr=Inherit: Inherit via back propagation  PCopyOutMin=[]  PCopyOutMax=[]  NCopyOutDataTypeStr=Inherit: Inherit via back propagation  NCopyOutMin=[]  NCopyOutMax=[]  IntegratorContinuousStateAttributes=''  IntegratorStateMustResolveToSignalObject=off  IntegratorRTWStateStorageClass=Auto  FilterContinuousStateAttributes=''  FilterStateMustResolveToSignalObject=off  FilterRTWStateStorageClass=Auto  ParallelPVariant=InternalParameters  IdealPVariant=Disabled  IVariant=InternalParameters  DVariant=Disabled  IntegratorVariant=Continuous  SatVariant=Disabled  AWVariant=Passthrough  PCopyVariant=Disabled  TRVariant=Disabled  FdbkBlocksVariant=Forward  IdealPFdbkVariant=Disabled  SatFdbkVariant=Disabled  DerivativeFilterVariant=Disabled  NVariant=Disabled  NCopyVariant=Disabled_SignalSpec  FilterICVariant=Disabled  IntegratorICVariant=InternalICs  ExternalResetVariant=Disabled  TRSumVariant=Passthrough  SumFdbkVariant=Disabled  SumVariant=Sum_PI  TsampFilterVariant=InternalTs  TsampNgainVariant=Passthrough  TsampIntegralVariant=Disabled_SignalSpec  ExternalSaturationOutDataTypeStr=Inherit: Same as second input  DerivativeSourceVariant=Disabled  PreIntVariant=InternalPreInt
  Scope : Scope  NumInputPorts=3
      settings: ActiveDisplayYMinimum=237.40854742566631  ActiveDisplayYMaximum=324.6469636585125
  Sistema electrico del motor : Subsystem
  Sum : Sum  Inputs=|+-
  Sum1 : Sum  Inputs=|+-
  k_T : Gain  Gain=Kt
  w4 : Outport
  wires:
  k_T/1 -> Sum1/1  "Torque"
  Sum/1 -> PID Controller/1  "Error de Velocidad"
  MATLAB Function/1(T_a) -> Sum1/2  "Torque negativo"
  1/J/1 -> Integrator/1
  Constant/1 -> MATLAB Function/2(kQ)
  Sum1/1 -> 1/J/1
  Integrator/1 -> w4/1, Scope/3, MATLAB Function/1(omega), Sistema electrico del motor/2(Velocidad), Sum/2  "Velocidad"
  Constant1/1 -> MATLAB Function/3(b)
  r_w4/1 -> Scope/2, Sum/1  "Referencia de Velocidad"
  Sistema electrico del motor/1(i) -> k_T/1, Scope/1  "Corriente"
  PID Controller/1 -> Gain/1
  Gain/1 -> Sistema electrico del motor/1(r_i)

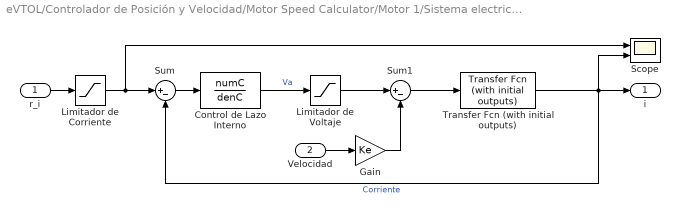
== system eVTOL/Controlador de Posición y Velocidad/Motor Speed Calculator/Motor 1/Sistema electrico del motor ==
  r_i : Inport
  Velocidad : Inport  Port=2
  Control de Lazo Interno : TransferFcn  Numerator=numC  Denominator=denC
  Gain : Gain  Gain=Ke
  Limitador de Corriente : Saturate  UpperLimit=200  LowerLimit=0  LinearizeAsGain=off
  Limitador de Voltaje : Saturate  UpperLimit=53.3  LowerLimit=0  LinearizeAsGain=off
  Scope : Scope  NumInputPorts=2
      settings: ActiveDisplayYMinimum=29.972492069722065  ActiveDisplayYMaximum=56.693249938370563
  Sum : Sum  Inputs=|+-
  Sum1 : Sum  Inputs=|+-
  Transfer Fcn (with initial outputs) : simulink_extras/Additional Linear/Transfer Fcn (with initial outputs)  N=[1]  D="[La  Ra]"  Y0=20  U0=0
  i : Outport
  wires:
  r_i/1 -> Limitador de Corriente/1
  Transfer Fcn (with initial outputs)/1 -> Sum/2, i/1, Scope/2  "Corriente"
  Control de Lazo Interno/1 -> Limitador de Voltaje/1  "Va"
  Sum/1 -> Control de Lazo Interno/1
  Limitador de Corriente/1 -> Sum/1, Scope/1
  Limitador de Voltaje/1 -> Sum1/1
  Velocidad/1 -> Gain/1
  Gain/1 -> Sum1/2
  Sum1/1 -> Transfer Fcn (with initial outputs)/1

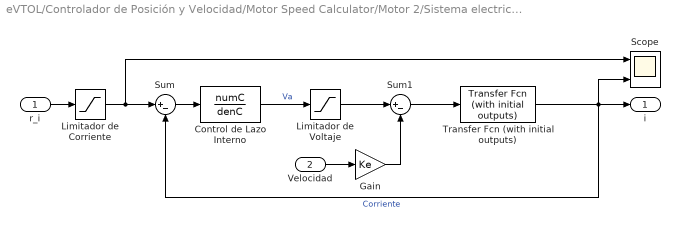
== system eVTOL/Controlador de Posición y Velocidad/Motor Speed Calculator/Motor 2/Sistema electrico del motor ==
  r_i : Inport
  Velocidad : Inport  Port=2
  Control de Lazo Interno : TransferFcn  Numerator=numC  Denominator=denC
  Gain : Gain  Gain=Ke
  Limitador de Corriente : Saturate  UpperLimit=200  LowerLimit=0  LinearizeAsGain=off
  Limitador de Voltaje : Saturate  UpperLimit=53.3  LowerLimit=0  LinearizeAsGain=off
  Scope : Scope  NumInputPorts=2
      settings: ActiveDisplayYMinimum=-32.070178200962914  ActiveDisplayYMaximum=95.013848575218262
  Sum : Sum  Inputs=|+-
  Sum1 : Sum  Inputs=|+-
  Transfer Fcn (with initial outputs) : simulink_extras/Additional Linear/Transfer Fcn (with initial outputs)  N=[1]  D="[La  Ra]"  Y0=20  U0=0
  i : Outport
  wires:
  r_i/1 -> Limitador de Corriente/1
  Transfer Fcn (with initial outputs)/1 -> Sum/2, i/1, Scope/2  "Corriente"
  Control de Lazo Interno/1 -> Limitador de Voltaje/1  "Va"
  Sum/1 -> Control de Lazo Interno/1
  Limitador de Corriente/1 -> Sum/1, Scope/1
  Limitador de Voltaje/1 -> Sum1/1
  Velocidad/1 -> Gain/1
  Gain/1 -> Sum1/2
  Sum1/1 -> Transfer Fcn (with initial outputs)/1

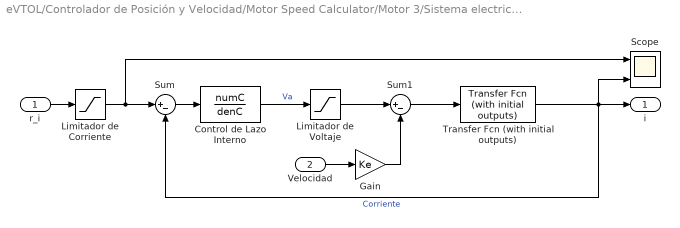
== system eVTOL/Controlador de Posición y Velocidad/Motor Speed Calculator/Motor 3/Sistema electrico del motor ==
  r_i : Inport
  Velocidad : Inport  Port=2
  Control de Lazo Interno : TransferFcn  Numerator=numC  Denominator=denC
  Gain : Gain  Gain=Ke
  Limitador de Corriente : Saturate  UpperLimit=200  LowerLimit=0  LinearizeAsGain=off
  Limitador de Voltaje : Saturate  UpperLimit=53.3  LowerLimit=0  LinearizeAsGain=off
  Scope : Scope  NumInputPorts=2
      settings: ActiveDisplayYMinimum=-32.070178200962914  ActiveDisplayYMaximum=95.013848575218262
  Sum : Sum  Inputs=|+-
  Sum1 : Sum  Inputs=|+-
  Transfer Fcn (with initial outputs) : simulink_extras/Additional Linear/Transfer Fcn (with initial outputs)  N=[1]  D="[La  Ra]"  Y0=20  U0=0
  i : Outport
  wires:
  r_i/1 -> Limitador de Corriente/1
  Transfer Fcn (with initial outputs)/1 -> Sum/2, i/1, Scope/2  "Corriente"
  Control de Lazo Interno/1 -> Limitador de Voltaje/1  "Va"
  Sum/1 -> Control de Lazo Interno/1
  Limitador de Corriente/1 -> Sum/1, Scope/1
  Limitador de Voltaje/1 -> Sum1/1
  Velocidad/1 -> Gain/1
  Gain/1 -> Sum1/2
  Sum1/1 -> Transfer Fcn (with initial outputs)/1

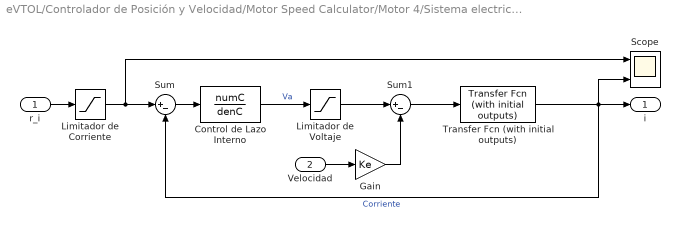
== system eVTOL/Controlador de Posición y Velocidad/Motor Speed Calculator/Motor 4/Sistema electrico del motor ==
  r_i : Inport
  Velocidad : Inport  Port=2
  Control de Lazo Interno : TransferFcn  Numerator=numC  Denominator=denC
  Gain : Gain  Gain=Ke
  Limitador de Corriente : Saturate  UpperLimit=200  LowerLimit=0  LinearizeAsGain=off
  Limitador de Voltaje : Saturate  UpperLimit=53.3  LowerLimit=0  LinearizeAsGain=off
  Scope : Scope  NumInputPorts=2
      settings: ActiveDisplayYMinimum=-32.070178200962914  ActiveDisplayYMaximum=95.013848575218262
  Sum : Sum  Inputs=|+-
  Sum1 : Sum  Inputs=|+-
  Transfer Fcn (with initial outputs) : simulink_extras/Additional Linear/Transfer Fcn (with initial outputs)  N=[1]  D="[La  Ra]"  Y0=20  U0=0
  i : Outport
  wires:
  r_i/1 -> Limitador de Corriente/1
  Transfer Fcn (with initial outputs)/1 -> Sum/2, i/1, Scope/2  "Corriente"
  Control de Lazo Interno/1 -> Limitador de Voltaje/1  "Va"
  Sum/1 -> Control de Lazo Interno/1
  Limitador de Corriente/1 -> Sum/1, Scope/1
  Limitador de Voltaje/1 -> Sum1/1
  Velocidad/1 -> Gain/1
  Gain/1 -> Sum1/2
  Sum1/1 -> Transfer Fcn (with initial outputs)/1

== matlab function eVTOL/Controlador de Posición y Velocidad/Motor Speed Calculator/Motor 4/MATLAB Function ==
  data: omega input; T_a output; kQ input; b input
function T_a = fcn(omega,kQ, b)
T_a=(omega^2)*kQ+b*omega; 
end

== matlab function eVTOL/Controlador de Posición y Velocidad/Motor Speed Calculator/Controlador de Actitud/MATLAB Function ==
  data: psi input; fx_b output; fy_b output; Fy_ref input; Fx_ref input
function [fx_b,fy_b] = fcn(psi,Fy_ref,Fx_ref)
% Rotación de Fuerzas (World -> Heading Frame)
    % Proyectamos la fuerza deseada en la dirección actual de la nariz
    fx_b = Fx_ref * cos(psi) + Fy_ref * sin(psi);
    fy_b = -Fx_ref * sin(psi) + Fy_ref * cos(psi);

== matlab function eVTOL/Controlador de Posición y Velocidad/Motor Speed Calculator/MATLAB Function ==
  data: omega1_ref output; T input; M_tita input; omega2_ref output; KF parameter; l parameter; M_phi input; M_psi input; omega3_ref output; omega4_ref output
function [omega1_ref, omega2_ref, omega3_ref, omega4_ref] = omega_calculator(T, M_tita, KF, l, M_phi, M_psi)
    % Entradas:
    % T: Empuje Total (N)
    % M_tita: Momento Pitch (N.m) -> Nariz Arriba/Abajo
    % KF: Coeficiente de empuje (N / (rad/s)^2)
    % l: Distancia del centro al eje del motor (brazo de momento directo)
    % M_phi: Momento Roll (N.m) -> Alabeo Izquierda/Derecha
    % M_psi: Momento Yaw (N.m) -> Guiñada (Giro sobre eje Z)
    
    % --- 1. Cálculo de componentes de Fuerza ---
    % Cada término calcula cuánta fuerza necesita aportar cada motor individualmente
    
    f_thrust = T / 4;              % Empuje base por motor
    f_pitch = M_tita / (4 * l);   % Fuerza para Pitch (4 porque los 4 motores trabajan)
    f_roll   = M_phi  / (4 * l);   % Fuerza para Roll
    f_yaw    = M_psi  / 4;         % Fuerza equivalente para Yaw (asumiendo acople directo)

    % --- 2. Mezclador (Mixer) para Cuadrado ---
    % Asumiendo numeración estándar:
    % 1: Frente-Izquierda
    % 2: Frente-Derecha
    % 3: Atrás-Derecha
    % 4: Atrás-Izquierda
    
    % SIGNOS (Ajustar según tu sentido de giro de motores):
    % Pitch (+): Levantar nariz -> Motores Frente (1,2) suben, Atrás (3,4) bajan.
    % Roll (+): Caer a derecha -> Motores Izq (1,4) suben, Der (2,3) bajan.
    % Yaw (+): Giro horario -> Motores CCW suben, CW bajan.

    T1 = f_thrust - f_pitch + f_roll - f_yaw; % Frente-Izq
    T2 = f_thrust - f_pitch - f_roll + f_yaw; % Frente-Der
    T3 = f_thrust + f_pitch - f_roll - f_yaw; % Atrás-Der
    T4 = f_thrust + f_pitch + f_roll + f_yaw; % Atrás-Izq

    % --- 3. Saturación (Física: hélices no empujan negativo) ---
    T1 = max(T1, 0);
    T2 = max(T2, 0);
    T3 = max(T3, 0);
    T4 = max(T4, 0);

    % --- 4. Conversión a Velocidad Angular ---
    omega1_ref = sqrt(T1 / KF);
    omega2_ref = sqrt(T2 / KF);
    omega3_ref = sqrt(T3 / KF);
    omega4_ref = sqrt(T4 / KF);
end

== matlab function eVTOL/Controlador de Posición y Velocidad/Motor Speed Calculator/Motor 1/MATLAB Function ==
  data: omega input; T_a output; kQ input; b input
function T_a = fcn(omega,kQ, b)
T_a=(omega^2)*kQ+b*omega; 
end

== matlab function eVTOL/Controlador de Posición y Velocidad/Motor Speed Calculator/Motor 2/MATLAB Function ==
  data: omega input; T_a output; kQ input; b input
function T_a = fcn(omega,kQ, b)
T_a=(omega^2)*kQ+b*omega; 
end

== matlab function eVTOL/Controlador de Posición y Velocidad/Motor Speed Calculator/MATLAB Function1 ==
  data: omega1 input; T1 output; omega2 input; omega3 input; omega4 input; T2 output; T3 output; KF parameter; l_palanca parameter; T4 output; Mx output; My output; Mz output; velocidades_angulares input; J_xz parameter
function [T1, T2, T3, T4, Mx,My,Mz] = T_calculator(omega1, omega2, omega3, omega4, KF, l_palanca, velocidades_angulares,J_xz)
    % Entradas:
    % omegas: Velocidades angulares de cada motor (rad/s)
    % KF: Coeficiente de empuje (N / (rad/s)^2)
    % KM: Coeficiente de momento/drag (N.m / (rad/s)^2) -> NUEVO PARA YAW
    % l_palanca: Distancia del centro al motor (m)

    % 1. Calcular Empujes individuales (Thrust)
    T1 = KF * omega1^2;
    T2 = KF * omega2^2;
    T3 = KF * omega3^2;
    T4 = KF * omega4^2;
    
    % 2. Calcular Momentos (Torques) sobre el cuerpo
    % Asumiendo la misma numeración cuadrada del mixer anterior:
    % 1: Frente-Izq, 2: Frente-Der, 3: Atrás-Der, 4: Atrás-Izq
    I = diag([J_xz,J_xz,J_xz]);   
    tau_gyro = cross(velocidades_angulares, I*velocidades_angulares);   % omega x (I omega)


    % Momento de ROLL (Mx) - Eje X - PHI
    % Diferencia entre lado Izquierdo (1,4) y Derecho (2,3)
    % Si Izq empuja más, genera momento positivo (rolido a derecha)
    Mx = l_palanca * ((T1 + T4) - (T2 + T3))-tau_gyro(1);

    % Momento de PITCH (My) - Eje Y - TITA
    % Diferencia entre Frente (1,2) y Atrás (3,4)
    % Si Frente empuja más, nariz sube (Pitch positivo)
    My = l_palanca * (-(T1 + T2) +(T3 + T4))-tau_gyro(2);

    % Momento de YAW (Mz) - Eje Z
    % Producido por el par reactivo de las hélices (Drag).
    % Depende de qué motores giran horario (CW) y antihorario (CCW).
    % Supuesto estándar: 1,3 giran CW (-) y 2,4 giran CCW (+)
    %Mz = 1 * (-omega1^2 + omega2^2 - omega3^2 + omega4^2);
    Mz=0;
end

== matlab function eVTOL/Controlador de Posición y Velocidad/Motor Speed Calculator/MATLAB Function2 ==
  data: Fx output; Fy output; T1 input; T2 input; T3 input; T4 input; phi input; tita input; psi input; Vx input; Vy input; Vz input; Fz output; m parameter
function [Fx, Fy, Fz] = calc_fuerza(T1, T2, T3, T4, phi, tita, psi, Vx, Vy, Vz, m)
    % Constantes Aerodinámicas
    Cdx = 1;
    Cdy = 1; % Agregado para eje lateral
    Cdz = 2;
    S = 1;
    rho = 1.225;
    g = 9.81;

% --- 1. Vector Empuje en Coordenadas Cuerpo (Body) ---
    % El empuje siempre apunta en el eje Z positivo del Dron (hacia "su" arriba)
    U_total = T1 + T2 + T3 + T4;
    F_body = [0; 0; U_total];

    % 2. Fuerzas de Drag (Resistencia del aire)
    % 0.5 * rho * S * Cd * V^2 * sign(V)
    Dx = 0.5 * rho * S * Cdx * Vx^2 * sign(Vx);
    Dy = 0.5 * rho * S * Cdy * Vy^2 * sign(Vy);
    Dz = 0.5 * rho * S * Cdz * Vz^2 * sign(Vz);

% --- 3. Matriz de Rotación R_IB (Body -> Inertial/Mundo) ---
    % Secuencia Z-Y-X estándar para ENU
    
    % Pre-cálculo de senos y cosenos
    cph = cos(phi);  sph = sin(phi);   % Roll
    cth = cos(tita); sth = sin(tita);  % Pitch
    cps = cos(psi);  sps = sin(psi);   % Yaw

    % Matriz de Rotación por ejes (Más seguro que escribir la fórmula final)
    % Rotación en X (Roll)
    Rx = [1   0    0;
          0  cph -sph;
          0  sph  cph];
      
    % Rotación en Y (Pitch) - OJO: En ENU, Pitch positivo baja la nariz o la sube
    % dependiendo de tu convención. Esta matriz asume Pitch+ = Nariz Arriba.
    Ry = [ cth  0  sth;
            0   1   0;
          -sth  0  cth];

    % Rotación en Z (Yaw)
    Rz = [cps -sps  0;
          sps  cps  0;
           0    0   1];

    % Matriz Completa: R_mundo_cuerpo = Rz * Ry * Rx
    R_IB = Rz * Ry * Rx;

    % --- 4. Rotar el Empuje al Mundo ---
    % F_mundo = R_IB * F_body
    F_inertial = R_IB * F_body; 

    % Extraemos componentes rotadas
    Tx = F_inertial(1);
    Ty = F_inertial(2);
    Tz = F_inertial(3);

    % 4. Sumatoria de Fuerzas Finales
    Fx = Tx - Dx;
    Fy = Ty - Dy;
    Fz = Tz - m*g - Dz; 
end
